simulink model "dinamicaralik"  (R2023b)
settings: Solver=ode45  StartTime=0.0  StopTime=50  FixedStep=0.0001  RelTol=1e-3
InitFcn:
  | Kpz = 0.3 ;
  | KIz = 0;
  | 
  | bh = 0.010290;  % batan hacim m^3
  | m = 10.5     ;  % aracın kütlesi kg
  | g = 9.81     ;  % yer çekimi ivmesi
  | p = 1000     ; % kg / m^3 yogunluk
  | W = m*g      ;  % aracın agırlıgı N
  | B = p*g*bh   ;  % Kaldırma kuvveti  N
  | 
  | xg = 0 ; % rgid body frame e göre ağırlık merkzi kordinatları
  | yg = 0 ;
  | zg = 0.02 ;
  | 
  | Ix = 0.1011 ; % kg *  m ^2
  | Iy = 0.1159 ;
  | Iz = 0.1615 ;
  | 
  | thrustCoefficient = 50/21.5 ;
  | 
  | % Add mass parametreleri
  | Xu_dot = -5.5;   % Surge direction
  | Yv_dot = -12.7;  % Sway direction
  | Zw_dot = -14.57; % Heave direction
  | 
  | Kp_dot = -0.12;  % Roll moment
  | Mq_dot = -0.12;  % Pitch moment
  | Nr_dot = -0.12;  % Yaw moment
  | 
  | % Linear Damping Values (Doğrusal Sönümleme Katsayıları)
  | Xu = -4.03;   % Ns/m
  | Yv = -6.22;   % Ns/m
  | Zw = -5.18;   % Ns/m
  | Kp = -0.07;   % Ns/rad
  | Mq = -0.07;   % Ns/rad
  | Nr = -0.07;   % Ns/rad
  | 
  | % Quadratic Damping Values (Doğrusal Olmayan Sönümleme Katsayıları)
  | Xuu = -18.18;  % Ns^2/m^2
  | Yvv = -21.66;  % Ns^2/m^2
  | Zww = -36.99;  % Ns^2/m^2
  | Kpp = -1.55;   % Ns^2/rad^2
  | Mqq = -1.55;   % Ns^2/rad^2
  | Nrr = -1.55;   % Ns^2/rad^2
undefined symbols (not defined in the file or in its folder): smiData, X, Y, Z
libraries: slpidlib x41, nesl_utility x14, sm_lib x12
(part 2 of 7)

== system dinamicaralik/SİM1 ==
  velo NED : Inport
  6-DOF Joint : sm_lib/Joints/6-DOF Joint  JointMode=Normal  SenseConstraintForce=off  SenseConstraintForceX=off  SenseConstraintForceY=off  SenseConstraintForceZ=off  SenseConstraintTorque=off  SenseConstraintTorqueX=off  SenseConstraintTorqueY=off  SenseConstraintTorqueZ=off  SenseTotalForce=off  SenseTotalForceX=off  SenseTotalForceY=off  SenseTotalForceZ=off  SenseTotalTorque=off  SenseTotalTorqueX=off  SenseTotalTorqueY=off  SenseTotalTorqueZ=off  CompositeWrenchDir=FollowerOnBase  CompositeWrenchFrame=BaseFrame  PxEquilibriumPosition=0  PxEquilibriumPositionUnits=m  PxSpringStiffness=0  PxSpringStiffnessUnits=N/m  PxDampingCoefficient=0  PxDampingCoefficientUnits=N/(m/s)  PxTorqueActuationMode=ComputedTorque  PxMotionActuationMode=InputMotion  PxSensePosition=off  PxSenseVelocity=off  PxSenseAcceleration=off  PxSenseTorqueForce=off  PxSenseLowerLimitTorqueForce=off  PxSenseUpperLimitTorqueForce=off  PxLowerLimitSpecify=off  PxLowerLimitBound=-1  PxLowerLimitBoundUnits=m  PxLowerLimitStiffness=1e6  PxLowerLimitStiffnessUnits=N/m  PxLowerLimitDamping=1e3  PxLowerLimitDampingUnits=N/(m/s)  PxLowerLimitTransitionRegionWidth=1e-4  PxLowerLimitTransitionRegionWidthUnits=m  PxUpperLimitSpecify=off  PxUpperLimitBound=1  PxUpperLimitBoundUnits=m  PxUpperLimitStiffness=1e6  PxUpperLimitStiffnessUnits=N/m  PxUpperLimitDamping=1e3  PxUpperLimitDampingUnits=N/(m/s)  PxUpperLimitTransitionRegionWidth=1e-4  PxUpperLimitTransitionRegionWidthUnits=m  PxPositionTargetSpecify=off  PxPositionTargetPriority=High  PxPositionTargetValue=0  PxPositionTargetValueUnits=m  PxVelocityTargetSpecify=off  PxVelocityTargetPriority=High  PxVelocityTargetValue=0  PxVelocityTargetValueUnits=m/s  PyEquilibriumPosition=0  PyEquilibriumPositionUnits=m  PySpringStiffness=0  PySpringStiffnessUnits=N/m  PyDampingCoefficient=0  PyDampingCoefficientUnits=N/(m/s)  PyTorqueActuationMode=ComputedTorque  PyMotionActuationMode=InputMotion  PySensePosition=off  PySenseVelocity=off  PySenseAcceleration=off  PySenseTorqueForce=off  PySenseLowerLimitTorqueForce=off  PySenseUpperLimitTorqueForce=off  PyLowerLimitSpecify=off  PyLowerLimitBound=-1  PyLowerLimitBoundUnits=m  PyLowerLimitStiffness=1e6  PyLowerLimitStiffnessUnits=N/m  PyLowerLimitDamping=1e3  PyLowerLimitDampingUnits=N/(m/s)  PyLowerLimitTransitionRegionWidth=1e-4  PyLowerLimitTransitionRegionWidthUnits=m  PyUpperLimitSpecify=off  PyUpperLimitBound=1  PyUpperLimitBoundUnits=m  PyUpperLimitStiffness=1e6  PyUpperLimitStiffnessUnits=N/m  PyUpperLimitDamping=1e3  PyUpperLimitDampingUnits=N/(m/s)  PyUpperLimitTransitionRegionWidth=1e-4  PyUpperLimitTransitionRegionWidthUnits=m  PyPositionTargetSpecify=off  PyPositionTargetPriority=High  PyPositionTargetValue=0  PyPositionTargetValueUnits=m  PyVelocityTargetSpecify=off  PyVelocityTargetPriority=High  PyVelocityTargetValue=0  PyVelocityTargetValueUnits=m/s  PzEquilibriumPosition=0  PzEquilibriumPositionUnits=m  PzSpringStiffness=0  PzSpringStiffnessUnits=N/m  PzDampingCoefficient=0  PzDampingCoefficientUnits=N/(m/s)  PzTorqueActuationMode=ComputedTorque  PzMotionActuationMode=InputMotion  PzSensePosition=off  PzSenseVelocity=off  PzSenseAcceleration=off  PzSenseTorqueForce=off  PzSenseLowerLimitTorqueForce=off  PzSenseUpperLimitTorqueForce=off  PzLowerLimitSpecify=off  PzLowerLimitBound=-1  PzLowerLimitBoundUnits=m  PzLowerLimitStiffness=1e6  PzLowerLimitStiffnessUnits=N/m  PzLowerLimitDamping=1e3  PzLowerLimitDampingUnits=N/(m/s)  PzLowerLimitTransitionRegionWidth=1e-4  PzLowerLimitTransitionRegionWidthUnits=m  PzUpperLimitSpecify=off  PzUpperLimitBound=1  PzUpperLimitBoundUnits=m  PzUpperLimitStiffness=1e6  PzUpperLimitStiffnessUnits=N/m  PzUpperLimitDamping=1e3  PzUpperLimitDampingUnits=N/(m/s)  PzUpperLimitTransitionRegionWidth=1e-4  PzUpperLimitTransitionRegionWidthUnits=m  PzPositionTargetSpecify=off  PzPositionTargetPriority=High  PzPositionTargetValue=0  PzPositionTargetValueUnits=m  PzVelocityTargetSpecify=off  PzVelocityTargetPriority=High  PzVelocityTargetValue=0  PzVelocityTargetValueUnits=m/s  SphEqPosRotationMethod=None  SphEqPosRotationAngleUnits=deg  SphEqPosRotationStandardAxis=+Z  SphEqPosRotationAngle=0  SphEqPosRotationArbitraryAxis=[0 0 1]  SphEqPosFollAlignAxisA=+X  SphEqPosBaseAlignAxisA=+Y  SphEqPosFollAlignAxisB=+Y  SphEqPosBaseAlignAxisB=+Z  SphEqPosRotationSequenceAxes=FollowerAxes  SphEqPosRotationSequence=XYX  SphEqPosRotationSequenceAngles=[0 0 0]  SphEqPosRotationSequenceAnglesUnits=deg  SphEqPosRotationMatrix=[1 0 0;0 1 0;0 0 1]  SphEqPosQuaternion=[1 0 0 0]  SphSpringStiffness=0  SphSpringStiffnessUnits=N*m/deg  SphDampingCoefficient=0  SphDampingCoefficientUnits=N*m/(deg/s)  SphActuateTorqueX=on  SphActuateTorqueY=on  SphActuateTorqueZ=on  SphActuateTorque=off  SphTorqueActuationMode=InputTorque  SphMotionActuationMode=ComputedMotion  SphActuationFrame=BaseFrame  SphSensePosition=off  SphSenseVelocityX=off  SphSenseVelocityY=off  SphSenseVelocityZ=off  SphSenseVelocity=off  SphSenseAccelerationX=off  SphSenseAccelerationY=off  SphSenseAccelerationZ=off  SphSenseAcceleration=off  SphSenseTorqueX=off  SphSenseTorqueY=off  SphSenseTorqueZ=off  SphSenseTorqueForce=off  SphSenseLowerLimitTorqueMag=off  SphSenseUpperLimitTorqueMag=off  SphSensingFrame=BaseFrame  SphLowerLimitSpecify=off  SphLowerLimitBound=15  SphLowerLimitBoundUnits=deg  SphLowerLimitStiffness=1e4  SphLowerLimitStiffnessUnits=N*m/deg  SphLowerLimitDamping=10  SphLowerLimitDampingUnits=N*m/(deg/s)  SphLowerLimitTransitionRegionWidth=0.1  SphLowerLimitTransitionRegionWidthUnits=deg  SphUpperLimitSpecify=off  SphUpperLimitBound=45  SphUpperLimitBoundUnits=deg  SphUpperLimitStiffness=1e4  SphUpperLimitStiffnessUnits=N*m/deg  SphUpperLimitDamping=10  SphUpperLimitDampingUnits=N*m/(deg/s)  SphUpperLimitTransitionRegionWidth=0.1  SphUpperLimitTransitionRegionWidthUnits=deg  SphPositionTargetRotationMethod=None  SphPositionTargetRotationAngleUnits=deg  SphPositionTargetRotationStandardAxis=+Z  SphPositionTargetRotationAngle=0  SphPositionTargetRotationArbitraryAxis=[0 0 1]  SphPositionTargetFollAlignAxisA=+X  SphPositionTargetBaseAlignAxisA=+Y  SphPositionTargetFollAlignAxisB=+Y  SphPositionTargetBaseAlignAxisB=+Z  SphPositionTargetRotationSequenceAxes=FollowerAxes  SphPositionTargetRotationSequence=XYX  SphPositionTargetRotationSequenceAngles=[0 0 0]  SphPositionTargetRotationSequenceAnglesUnits=deg  SphPositionTargetRotationMatrix=[1 0 0;0 1 0;0 0 1]  SphPositionTargetQuaternion=[1 0 0 0]  SphPositionTargetSpecify=off  SphPositionTargetPriority=High  SphVelocityTargetValue=[0 0 0]  SphVelocityTargetValueUnits=deg/s  SphVelocityTargetSpecify=off  SphVelocityTargetPriority=High  SphVelocityTargetInFollowerFrame=on
  Cylindrical Solid : sm_lib/Body Elements/Cylindrical Solid  GraphicAmbientColor=[0.15 0.15 0.15 1.0]  BasedOnType=Density  CenterOfMass=[0 0 0]  CenterOfMassUnits=m  GraphicDiffuseColor=[0.5 0.5 0.5]  CylinderLength=1  CylinderLengthUnits=m  CylinderRadius=1  CylinderRadiusUnits=m  Density=1000  DensityUnits=kg/m^3  DoExposeReferenceFrame=on  GraphicEmissiveColor=[0.0 0.0 0.0 1.0]  ExportEntireGeometry=off  SerializedFrames=<Frames/>  MarkerShape=Sphere  MarkerSize=10  GraphicType=FromGeometry  InertiaType=CalculateFromGeometry  Mass=1  MassUnits=kg  MomentsOfInertia=[1 1 1]  MomentsOfInertiaUnits=kg*m^2  GraphicOpacity=1.0  ProductsOfInertia=[0 0 0]  ProductsOfInertiaUnits=kg*m^2  GraphicShininess=75  GraphicSpecularColor=[0.5 0.5 0.5 1.0]  GraphicVisPropType=SimpleVisualProperties
  Demux : Demux  Outputs=6
  Integrator : Integrator
  MechanismConfiguration : sm_lib/Utilities/Mechanism Configuration  UniformGravity=Constant  GravityVector=[0 -9.8 0]  GravityVectorUnits=m/s^2  LinearizationDelta=0.001  JointModeTransitionNonlinearIterations=2
  Simulink-PS Converter{,1..5} (6 alike) : nesl_utility/Simulink-PS Converter  PhysicalDomain=network_engine_domain  SubClassName=ps_input  LeftPortType=input  RightPortType=output  PseudoPeriodic=off  Frequencies=[]  NoiseDistribution=none  NoiseParameters=[]  Unit=1  AffineConversion=off  FilteringAndDerivatives=provide  SimscapeFilterOrder=1  InputFilterTimeConstant=0.001  UdotUserProvided=0
  Solver Configuration : nesl_utility/Solver Configuration  PhysicalDomain=network_engine_domain  SubClassName=solver  LeftPortType=input  RightPortType=generic  Tones=[]  Harmonics=[]  SimulateNoise=off  Profile=off  UseLocalSampling=off  EnableSwitchedLinearOptims=on  FrequencyDomain=off  UseCCode=off  RelTol=0.001  AbsTol=0.001  MinStep=1e-09  ToWorkspace=off  RevertToSquareIcSolve=off  NumHomotopyIterations=100  PhasorMode=off  PhasorModeNumHarmonics=1  ConsistencySolver=NEWTON_XTOL_AFTER_FTOL  IndexReductionMethod=DerivativeReplacement  DoDC=off  ResidualTolerance=1e-09  ConsistencyTolSource=GLOBAL  ConsistencyAbsTol=0.001  ConsistencyRelTol=0.001  ConsistencyTolFactor=0.001  UseLocalSolver=off  LocalSolverChoice=NE_BACKWARD_EULER_ADVANCER  ResolveIndetEquations=on  FunctionEvalNumThread=1  LocalSolverSampleTime=0.001  DoFixedCost=off  MaxNonlinIter=3  MaxModeIter=2  ComputeImpulses=off  ImpulseIterations=2  LinearAlgebra=auto  LinearAlgebraNumThread=0  EquationFormulation=NE_TIME_EF  DelaysMemoryBudget=1024  AutomaticFiltering=on  FilteringTimeConstant=0.001  PartitionStorageMethod=AS_NEEDED  PartitionMemoryBudget=1024  PartitionMethod=ROBUST  MultibodyUseLocalSolver=off  MultibodyLocalSolverChoice=ODE1  MultibodyLocalSolverSampleTime=0.001
  Transform : sm_lib/Frames and Transforms/Rigid Transform  TranslationMethod=Cartesian  TranslationStandardOffset=0  TranslationStandardOffsetUnits=m  TranslationStandardAxis=+Z  TranslationCartesianOffset=smiData.RigidTransform(37).translation  TranslationCartesianOffsetUnits=mm  TranslationROffset=0  TranslationROffsetUnits=m  TranslationZOffset=0  TranslationZOffsetUnits=m  TranslationThetaOffset=0  TranslationThetaOffsetUnits=deg  RotationMethod=ArbitraryAxis  RotationAngleUnits=rad  RotationStandardAxis=+Z  RotationAngle=0  RotationArbitraryAxis=[0,0,0]  FollAlignAxisA=+X  BaseAlignAxisA=+Y  FollAlignAxisB=+Y  BaseAlignAxisB=+Z  RotationSequenceAxes=FollowerAxes  RotationSequence=XYX  RotationSequenceAngles=[0 0 0]  RotationSequenceAnglesUnits=deg  RotationMatrix=[1 0 0;0 1 0;0 0 1]  Quaternion=[1 0 0 0]
  Transform1 : sm_lib/Frames and Transforms/Rigid Transform  TranslationMethod=Cartesian  TranslationStandardOffset=0  TranslationStandardOffsetUnits=m  TranslationStandardAxis=+Z  TranslationCartesianOffset=smiData.RigidTransform(37).translation  TranslationCartesianOffsetUnits=mm  TranslationROffset=0  TranslationROffsetUnits=m  TranslationZOffset=0  TranslationZOffsetUnits=m  TranslationThetaOffset=0  TranslationThetaOffsetUnits=deg  RotationMethod=ArbitraryAxis  RotationAngleUnits=rad  RotationStandardAxis=+Z  RotationAngle=0  RotationArbitraryAxis=[0,0,0]  FollAlignAxisA=+X  BaseAlignAxisA=+Y  FollAlignAxisB=+Y  BaseAlignAxisB=+Z  RotationSequenceAxes=FollowerAxes  RotationSequence=XYX  RotationSequenceAngles=[0 0 0]  RotationSequenceAnglesUnits=deg  RotationMatrix=[1 0 0;0 1 0;0 0 1]  Quaternion=[1 0 0 0]
  World : sm_lib/Frames and Transforms/World Frame
  wires:
  velo NED/1 -> Integrator/1
  Integrator/1 -> Demux/1
  Demux/1 -> Simulink-PS Converter/1
  Demux/2 -> Simulink-PS Converter1/1
  Demux/3 -> Simulink-PS Converter2/1
  Demux/4 -> Simulink-PS Converter3/1
  Demux/5 -> Simulink-PS Converter4/1
  Demux/6 -> Simulink-PS Converter5/1
  connections:
  Solver Configuration/RConn1 -- Transform/LConn1 -- MechanismConfiguration/RConn1 -- World/RConn1
  Simulink-PS Converter/RConn1 -- 6-DOF Joint/LConn2
  Simulink-PS Converter1/RConn1 -- 6-DOF Joint/LConn3
  6-DOF Joint/LConn5 -- Simulink-PS Converter3/RConn1
  6-DOF Joint/LConn4 -- Simulink-PS Converter2/RConn1
  Simulink-PS Converter5/RConn1 -- 6-DOF Joint/LConn7
  Simulink-PS Converter4/RConn1 -- 6-DOF Joint/LConn6
  Transform/RConn1 -- 6-DOF Joint/LConn1
  Transform1/RConn1 -- Cylindrical Solid/RConn1
  6-DOF Joint/RConn1 -- Transform1/LConn1

== system dinamicaralik/Throttle & Manifold ==
  note: Air Intake Dynamics
  Throttle Ang. : Inport
  "Engine Speed, N" : Inport  Port=2
  0 <= theta <= 90 : Saturate  UpperLimit=90  LowerLimit=0
  "Atmospheric Pressure, Pa (bar)" : Constant  Value=1.0
  Intake Manifold : Subsystem
      settings: RTWMemSecFuncInitTerm=Default  RTWMemSecFuncExecute=Default  RTWMemSecDataConstants=Default  RTWMemSecDataInternal=Default  RTWMemSecDataParameters=Default
  Throttle : Subsystem
      settings: RTWMemSecFuncInitTerm=Default  RTWMemSecFuncExecute=Default  RTWMemSecDataConstants=Default  RTWMemSecDataInternal=Default  RTWMemSecDataParameters=Default
  Air charge : Outport  InitialOutput=0  VectorParamsAs1DForOutWhenUnconnected=off
  wires:
  "Atmospheric Pressure, Pa (bar)"/1 -> Throttle/3("Atmospheric Pressure, Pa (bar) ")
  Intake Manifold/1(Air charge) -> Air charge/1
  Intake Manifold/2("Manifold Pressure, Pm (bar)") -> Throttle/2("Manifold Pressure, Pm (bar)")
  "Engine Speed, N"/1 -> Intake Manifold/2(N (rad/sec))
  Throttle/1("Throttle Flow, mdot (g/s)") -> Intake Manifold/1(mdot Input (g/s))
  Throttle Ang./1 -> 0 <= theta <= 90/1
  0 <= theta <= 90/1 -> Throttle/1("Throttle Angle, theta (deg)")

== system dinamicaralik/Vehicle Dynamics ==
  Teng : Inport
  Tload : Inport  Port=2
  "Inverse Inertia, 1/J" : Gain  Gain=1/0.14  SaturateOnIntegerOverflow=on  OutDataTypeStr=Inherit: Same as input  ParamDataTypeStr=Inherit: Same as input
  Sum : Sum  Inputs=+-  InputSameDT=on  SaturateOnIntegerOverflow=on  OutDataTypeStr=Inherit: Same as first input
  w = T/J w0 = 209 rad/s : Integrator  InitialCondition=209.48
  N : Outport  InitialOutput=0  VectorParamsAs1DForOutWhenUnconnected=off
  wires:
  "Inverse Inertia, 1/J"/1 -> w = T/J w0 = 209 rad/s/1
  w = T/J w0 = 209 rad/s/1 -> N/1
  Sum/1 -> "Inverse Inertia, 1/J"/1
  Teng/1 -> Sum/1
  Tload/1 -> Sum/2

== system dinamicaralik/ned ile kinematik olmadan ==
  Input : Inport
  From : From  Commented=on  GotoTag=posNED
  divecont : Subsystem  Commented=on
  divecont1 : Subsystem
  Out1 : Outport
  Out2 : Outport  Port=2
  wires:
  From/1 -> divecont/1(In1)
  divecont/1(Out1) -> Out1/1
  divecont1/1(Out1) -> Out2/1
  Input/1 -> divecont1/1(Input)

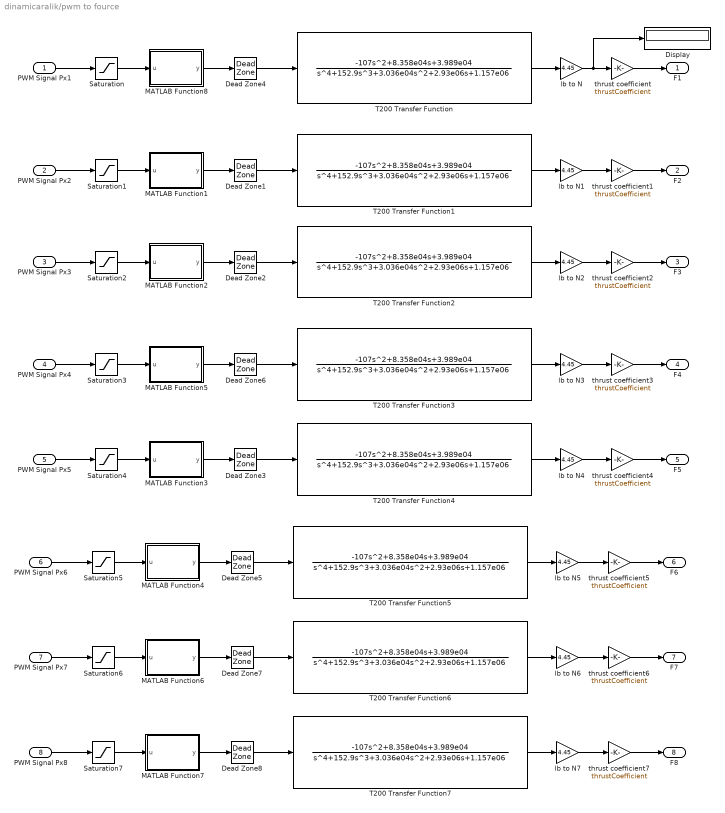
== system dinamicaralik/pwm to fource ==
  PWM Signal Px1 : Inport
  PWM Signal Px2 : Inport  Port=2
  PWM Signal Px3 : Inport  Port=3
  PWM Signal Px4 : Inport  Port=4
  PWM Signal Px5 : Inport  Port=5
  PWM Signal Px6 : Inport  Port=6
  PWM Signal Px7 : Inport  Port=7
  PWM Signal Px8 : Inport  Port=8
  Dead Zone{1..8} (8 alike) : DeadZone  LowerValue=-10  UpperValue=+10
  Display : Display
  MATLAB Function1 : MATLAB Function  TreatAsAtomicUnit=on
  MATLAB Function2 : MATLAB Function  TreatAsAtomicUnit=on
  MATLAB Function3 : MATLAB Function  TreatAsAtomicUnit=on
  MATLAB Function4 : MATLAB Function  TreatAsAtomicUnit=on
  MATLAB Function5 : MATLAB Function  TreatAsAtomicUnit=on
  MATLAB Function6 : MATLAB Function  TreatAsAtomicUnit=on
  MATLAB Function7 : MATLAB Function  TreatAsAtomicUnit=on
  MATLAB Function8 : MATLAB Function  TreatAsAtomicUnit=on
  Saturation{,1..7} (8 alike) : Saturate  UpperLimit=1900  LowerLimit=1100
  T200 Transfer Function{,1..7} (8 alike) : TransferFcn  Numerator="[-107  8.358e04  3.989e04]"  Denominator="[1 152.9  3.036e04  2.93e06  1.157e06]"
  lb to N{,1..7} (8 alike) : Gain  Gain=4.45
  thrust coefficient{,1..7} (8 alike) : Gain  Gain=thrustCoefficient
  F1 : Outport
  F2 : Outport  Port=2
  F3 : Outport  Port=3
  F4 : Outport  Port=4
  F5 : Outport  Port=5
  F6 : Outport  Port=6
  F7 : Outport  Port=7
  F8 : Outport  Port=8
  wires:
  PWM Signal Px1/1 -> Saturation/1
  MATLAB Function8/1(y) -> Dead Zone4/1
  T200 Transfer Function/1 -> lb to N/1
  Saturation/1 -> MATLAB Function8/1(u)
  Dead Zone4/1 -> T200 Transfer Function/1
  lb to N/1 -> Display/1, thrust coefficient/1
  thrust coefficient/1 -> F1/1
  Dead Zone1/1 -> T200 Transfer Function1/1
  T200 Transfer Function1/1 -> lb to N1/1
  lb to N1/1 -> thrust coefficient1/1
  MATLAB Function1/1(y) -> Dead Zone1/1
  Saturation1/1 -> MATLAB Function1/1(u)
  PWM Signal Px2/1 -> Saturation1/1
  thrust coefficient1/1 -> F2/1
  Dead Zone2/1 -> T200 Transfer Function2/1
  T200 Transfer Function2/1 -> lb to N2/1
  lb to N2/1 -> thrust coefficient2/1
  MATLAB Function2/1(y) -> Dead Zone2/1
  Saturation2/1 -> MATLAB Function2/1(u)
  PWM Signal Px3/1 -> Saturation2/1
  thrust coefficient2/1 -> F3/1
  PWM Signal Px6/1 -> Saturation5/1
  MATLAB Function4/1(y) -> Dead Zone5/1
  Dead Zone5/1 -> T200 Transfer Function5/1
  lb to N5/1 -> thrust coefficient5/1
  T200 Transfer Function5/1 -> lb to N5/1
  thrust coefficient5/1 -> F6/1
  Dead Zone6/1 -> T200 Transfer Function3/1
  T200 Transfer Function3/1 -> lb to N3/1
  MATLAB Function5/1(y) -> Dead Zone6/1
  Saturation3/1 -> MATLAB Function5/1(u)
  PWM Signal Px5/1 -> Saturation4/1
  Saturation4/1 -> MATLAB Function3/1(u)
  thrust coefficient4/1 -> F5/1
  MATLAB Function3/1(y) -> Dead Zone3/1
  Saturation5/1 -> MATLAB Function4/1(u)
  T200 Transfer Function4/1 -> lb to N4/1
  lb to N3/1 -> thrust coefficient3/1
  lb to N4/1 -> thrust coefficient4/1
  PWM Signal Px4/1 -> Saturation3/1
  thrust coefficient3/1 -> F4/1
  Dead Zone3/1 -> T200 Transfer Function4/1
  thrust coefficient7/1 -> F8/1
  PWM Signal Px8/1 -> Saturation7/1
  Dead Zone8/1 -> T200 Transfer Function7/1
  lb to N7/1 -> thrust coefficient7/1
  MATLAB Function7/1(y) -> Dead Zone8/1
  Dead Zone7/1 -> T200 Transfer Function6/1
  T200 Transfer Function6/1 -> lb to N6/1
  thrust coefficient6/1 -> F7/1
  T200 Transfer Function7/1 -> lb to N7/1
  MATLAB Function6/1(y) -> Dead Zone7/1
  PWM Signal Px7/1 -> Saturation6/1
  Saturation7/1 -> MATLAB Function7/1(u)
  lb to N6/1 -> thrust coefficient6/1
  Saturation6/1 -> MATLAB Function6/1(u)

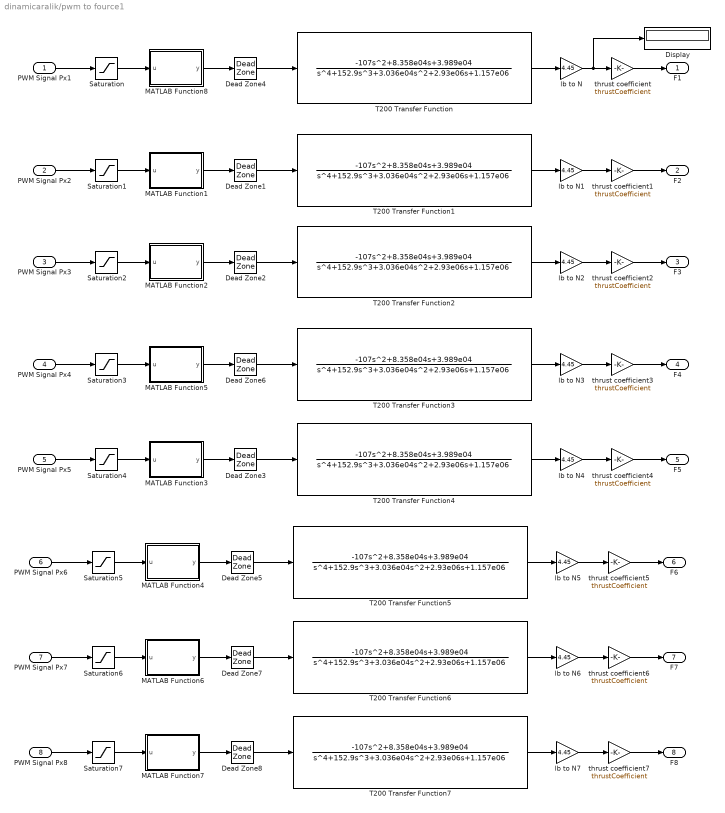
== system dinamicaralik/pwm to fource1 ==
  PWM Signal Px1 : Inport
  PWM Signal Px2 : Inport  Port=2
  PWM Signal Px3 : Inport  Port=3
  PWM Signal Px4 : Inport  Port=4
  PWM Signal Px5 : Inport  Port=5
  PWM Signal Px6 : Inport  Port=6
  PWM Signal Px7 : Inport  Port=7
  PWM Signal Px8 : Inport  Port=8
  Dead Zone{1..8} (8 alike) : DeadZone  LowerValue=-10  UpperValue=+10
  Display : Display
  MATLAB Function1 : MATLAB Function  TreatAsAtomicUnit=on
  MATLAB Function2 : MATLAB Function  TreatAsAtomicUnit=on
  MATLAB Function3 : MATLAB Function  TreatAsAtomicUnit=on
  MATLAB Function4 : MATLAB Function  TreatAsAtomicUnit=on
  MATLAB Function5 : MATLAB Function  TreatAsAtomicUnit=on
  MATLAB Function6 : MATLAB Function  TreatAsAtomicUnit=on
  MATLAB Function7 : MATLAB Function  TreatAsAtomicUnit=on
  MATLAB Function8 : MATLAB Function  TreatAsAtomicUnit=on
  Saturation{,1..7} (8 alike) : Saturate  UpperLimit=1900  LowerLimit=1100
  T200 Transfer Function{,1..7} (8 alike) : TransferFcn  Numerator="[-107  8.358e04  3.989e04]"  Denominator="[1 152.9  3.036e04  2.93e06  1.157e06]"
  lb to N{,1..7} (8 alike) : Gain  Gain=4.45
  thrust coefficient{,1..7} (8 alike) : Gain  Gain=thrustCoefficient
  F1 : Outport
  F2 : Outport  Port=2
  F3 : Outport  Port=3
  F4 : Outport  Port=4
  F5 : Outport  Port=5
  F6 : Outport  Port=6
  F7 : Outport  Port=7
  F8 : Outport  Port=8
  wires:
  PWM Signal Px1/1 -> Saturation/1
  MATLAB Function8/1(y) -> Dead Zone4/1
  T200 Transfer Function/1 -> lb to N/1
  Saturation/1 -> MATLAB Function8/1(u)
  Dead Zone4/1 -> T200 Transfer Function/1
  lb to N/1 -> Display/1, thrust coefficient/1
  thrust coefficient/1 -> F1/1
  Dead Zone1/1 -> T200 Transfer Function1/1
  T200 Transfer Function1/1 -> lb to N1/1
  lb to N1/1 -> thrust coefficient1/1
  MATLAB Function1/1(y) -> Dead Zone1/1
  Saturation1/1 -> MATLAB Function1/1(u)
  PWM Signal Px2/1 -> Saturation1/1
  thrust coefficient1/1 -> F2/1
  Dead Zone2/1 -> T200 Transfer Function2/1
  T200 Transfer Function2/1 -> lb to N2/1
  lb to N2/1 -> thrust coefficient2/1
  MATLAB Function2/1(y) -> Dead Zone2/1
  Saturation2/1 -> MATLAB Function2/1(u)
  PWM Signal Px3/1 -> Saturation2/1
  thrust coefficient2/1 -> F3/1
  PWM Signal Px6/1 -> Saturation5/1
  MATLAB Function4/1(y) -> Dead Zone5/1
  Dead Zone5/1 -> T200 Transfer Function5/1
  lb to N5/1 -> thrust coefficient5/1
  T200 Transfer Function5/1 -> lb to N5/1
  thrust coefficient5/1 -> F6/1
  Dead Zone6/1 -> T200 Transfer Function3/1
  T200 Transfer Function3/1 -> lb to N3/1
  MATLAB Function5/1(y) -> Dead Zone6/1
  Saturation3/1 -> MATLAB Function5/1(u)
  PWM Signal Px5/1 -> Saturation4/1
  Saturation4/1 -> MATLAB Function3/1(u)
  thrust coefficient4/1 -> F5/1
  MATLAB Function3/1(y) -> Dead Zone3/1
  Saturation5/1 -> MATLAB Function4/1(u)
  T200 Transfer Function4/1 -> lb to N4/1
  lb to N3/1 -> thrust coefficient3/1
  lb to N4/1 -> thrust coefficient4/1
  PWM Signal Px4/1 -> Saturation3/1
  thrust coefficient3/1 -> F4/1
  Dead Zone3/1 -> T200 Transfer Function4/1
  thrust coefficient7/1 -> F8/1
  PWM Signal Px8/1 -> Saturation7/1
  Dead Zone8/1 -> T200 Transfer Function7/1
  lb to N7/1 -> thrust coefficient7/1
  MATLAB Function7/1(y) -> Dead Zone8/1
  Dead Zone7/1 -> T200 Transfer Function6/1
  T200 Transfer Function6/1 -> lb to N6/1
  thrust coefficient6/1 -> F7/1
  T200 Transfer Function7/1 -> lb to N7/1
  MATLAB Function6/1(y) -> Dead Zone7/1
  PWM Signal Px7/1 -> Saturation6/1
  Saturation7/1 -> MATLAB Function7/1(u)
  lb to N6/1 -> thrust coefficient6/1
  Saturation6/1 -> MATLAB Function6/1(u)
